simulink model "chopper_dc"  (R2018a)
settings: Solver=VariableStepAuto  StartTime=0.0  StopTime=2  RelTol=1e-3
libraries: powerlib x12
settings Model: Creator=user  LastModifiedBy=user
settings SolverCC: ZeroCrossAlgorithm=Adaptive
settings DebuggingCC: MaxConsecutiveZCsMsg=none

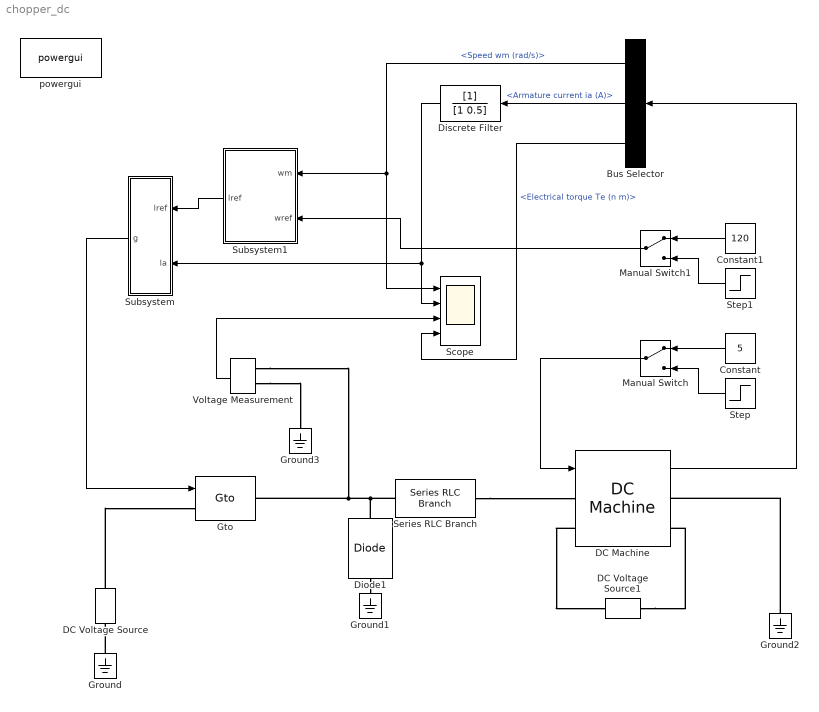
== system chopper_dc ==
  Bus Selector : BusSelector  OutputSignals=Speed wm (rad/s),Armature current ia (A),Electrical torque Te (n m)
  Constant : Constant  Value=5
  Constant1 : Constant  Value=120
  DC Machine : powerlib/Machines/DC Machine  PresetModel=No  MechanicalLoad=Torque TL  FieldType=Wound  ShowDetailedParameters=on  MeasurementBus=off  RLa=[0.5 0.01]  RLf=[240 120]  Laf=1.234  MachineConstant=Torque constant (N.m/A)  Ke=1.8  Kt=1.8  J=0.05  Bm=0.01  Tf=0  w0=1  Ifinit=1  TsPowergui=0  TsBlock=-1
  DC Voltage Source : powerlib/Electrical Sources/DC Voltage Source  Amplitude=280  Measurements=None
  DC Voltage Source1 : powerlib/Electrical Sources/DC Voltage Source  Amplitude=240  Measurements=None
  Diode1 : powerlib/Power Electronics/Diode  Ron=0.001  Lon=0  Vf=0.8  IC=0  UseSnubber=0  Rs=0  Cs=0  Measurements=off
  Discrete Filter : DiscreteFilter
  Ground{,1..3} (4 alike) : powerlib/Elements/Ground  LConnTagsString=a
  Gto : powerlib/Power Electronics/Gto  Ron=0.05  Lon=0  Vf=1  Tf=10e-6  Tt=20e-6  IC=0  Rs=1e5  Cs=inf  Measurements=off
      settings: SourceProductName=Simscape Power Systems  SourceProductBaseCode=PS
  Manual Switch : ManualSwitch
  Manual Switch1 : ManualSwitch
  Scope : Scope  NumInputPorts=4
  Series RLC Branch : powerlib/Elements/Series RLC Branch  LConnTagsString=__new0  RConnTagsString=__new0  BranchType=L  Resistance=1  Inductance=1e-3  SetiL0=off  InitialCurrent=0  Capacitance=1e-6  Setx0=off  InitialVoltage=0  Measurements=None
  Step : Step  SampleTime=0
  Step1 : Step  SampleTime=0
  Subsystem : Subsystem  mask{h=2}
      mask prompts: h "Hysteresis bamd (A)"
  Subsystem1 : Subsystem  mask{Kp=1.6, Ki=16, Ilim=30}
      mask prompts: Kp "Proportional gain (Kp)"; Ki "Integral gain (Ki)"; Ilim "Current limit (A)"
  Voltage Measurement : powerlib/Measurements/Voltage Measurement  PhasorSimulation=off  OutputType=Complex  PSBequivalent=0
  powergui : powerlib/powergui  Priority=1  SimulationMode=Continuous  SampleTime=50e-6  frequency=60  Iterations=50  frequencyindice=0  Pbase=100e6  ErrMax=1e-4  UnitsV=kV  UnitsW=MW  buscounter=0  FunctionMessages=off  echomessages=off  EnableUseOfTLC=off  CurrentSourceSwitches=off  DisableSnubberDevices=off  DisableRonSwitches=off  DisableVfSwitches=off  DisplayEquations=off  SolverType=Tustin/Backward Euler (TBE)  Interpol=off  ExternalGateDelay=off  methode=off  Ts=100  x0status=blocks  SPID=on  SwTol=0  HookPort=off  RestoreLinks=warning  ResistiveCurrentMeasurement=off  Frange=[0:2:500]  Ylog=off  Xlog=on  ShowGrid=off  save=off  variable=ZData  structure=0  ZoomFFT=off  StartTime=0.0  cycles=1  DisplayStyle=1  fundamental=60  FreqAxis=off  MaxFrequency=1000  frequencyindicesteady=1  RmsSteady=1  display=off
  wires:
  Constant/1 -> Manual Switch/1
  Step/1 -> Manual Switch/2
  Constant1/1 -> Manual Switch1/1
  Step1/1 -> Manual Switch1/2
  DC Machine/1 -> Bus Selector/1
  Voltage Measurement/1 -> Scope/3
  Discrete Filter/1 -> Subsystem/2(la), Scope/2
  Bus Selector/2 -> Discrete Filter/1  "<Armature current ia (A)>"
  Subsystem1/1(lref) -> Subsystem/1(lref)
  Subsystem/1("g ") -> Gto/1
  Manual Switch1/1 -> Subsystem1/2(wref)
  Bus Selector/1 -> Scope/1, Subsystem1/1(wm)  "<Speed wm (rad/s)>"
  Manual Switch/1 -> DC Machine/1
  Bus Selector/3 -> Scope/4  "<Electrical torque Te (n m)>"
  connections:
  Ground/LConn1 -- DC Voltage Source/LConn1
  DC Voltage Source/RConn1 -- Gto/LConn1
  Series RLC Branch/LConn1 -- Voltage Measurement/LConn1 -- Gto/RConn1 -- Diode1/RConn1
  Series RLC Branch/RConn1 -- DC Machine/LConn1
  DC Machine/LConn2 -- DC Voltage Source1/RConn1
  DC Voltage Source1/LConn1 -- DC Machine/RConn2
  Ground2/LConn1 -- DC Machine/RConn1
  Voltage Measurement/LConn2 -- Ground3/LConn1
  Diode1/LConn1 -- Ground1/LConn1

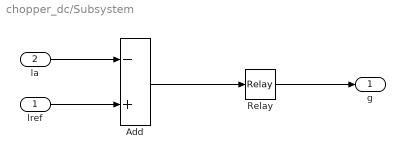
== system chopper_dc/Subsystem ==
  lref : Inport
  la : Inport  Port=2
  Add : Sum  Inputs=-+
  Relay : Relay  OnSwitchValue=h/2  OffSwitchValue=-h/2
  "g " : Outport  VectorParamsAs1DForOutWhenUnconnected=on
  wires:
  lref/1 -> Add/2
  Relay/1 -> "g "/1
  la/1 -> Add/1
  Add/1 -> Relay/1

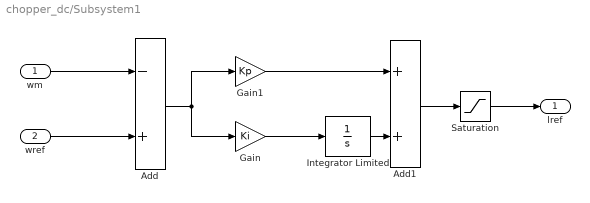
== system chopper_dc/Subsystem1 ==
  wm : Inport
  wref : Inport  Port=2
  Add : Sum  Inputs=-+
  Add1 : Sum
  Gain : Gain  Gain=Ki
  Gain1 : Gain  Gain=Kp
  Integrator Limited : Integrator  LimitOutput=on  UpperSaturationLimit=Ilim  LowerSaturationLimit=-Ilim
  Saturation : Saturate  UpperLimit=Ilim  LowerLimit=-Ilim
  lref : Outport  VectorParamsAs1DForOutWhenUnconnected=on
  wires:
  Add/1 -> Gain1/1, Gain/1
  Saturation/1 -> lref/1
  wref/1 -> Add/2
  wm/1 -> Add/1
  Gain1/1 -> Add1/1
  Integrator Limited/1 -> Add1/2
  Gain/1 -> Integrator Limited/1
  Add1/1 -> Saturation/1
